simulink model "interp_2D_flat_CLIP_last_index_true"  (R2017b)
settings: Solver=FixedStepAuto  StartTime=0.0  StopTime=10.0  FixedStep=0.1  RelTol=1e-3  EnableMultiTasking=on
settings Model: ExtModeAutoUpdateStatusClock=off  Creator=The MathWorks, Inc.  LastModifiedBy=hbourbou
settings DataIOCC: LimitDataPoints=on  SaveFormat=Array  SignalLoggingName=sigsOut
settings OptimizationCC: BooleanDataType=off  ExpressionDepthLimit=2147483647  InitFltsAndDblsToZero=on  LifeSpan=inf
settings DebuggingCC: SaveWithParameterizedLinksMsg=none  UnderspecifiedInitializationDetection=Classic  MergeDetectMultiDrivingBlocksExec=none  CheckExecutionContextPreStartOutputMsg=on  CheckExecutionContextRuntimeOutputMsg=on  SignalResolutionControl=TryResolveAllWithWarning  MultiTaskDSMMsg=warning  MultiTaskCondExecSysMsg=none  FcnCallInpInsideContextMsg=warning  StateNameClashWarn=warning  SFUnexpectedBacktrackingDiag=warning  SFNoUnconditionalDefaultTransitionDiag=warning  SFExecutionAtInitializationDiag=none
settings HardwareCC: ProdBitPerPointer=32  ProdBitPerSizeT=32  ProdBitPerPtrDiffT=32  ProdLargestAtomicFloat=None  ProdIntDivRoundTo=Undefined  ProdEndianess=Unspecified  ProdWordSize=32  ProdHWDeviceType=32-bit Generic  TargetUnknown=on
settings ModelReferenceCC: PropagateSignalLabelsOutOfModel=off
settings CodeAppCC: StateflowObjectComments=on
settings GRTTargetCC: TargetFcnLib=ansi_tfl_tmw.mat  TargetLangStandard=C89/C90 (ANSI)  GeneratePreprocessorConditionals=Disable all  CombineOutputUpdateFcns=off  GRTInterface=on
settings ConfigComp: CovMetricSettings=dw  CovHtmlReporting=on  CovSaveCumulativeToWorkspaceVar=on  CovSaveSingleToWorkspaceVar=on  CovExternalEMLEnable=off  CovSFcnEnable=off

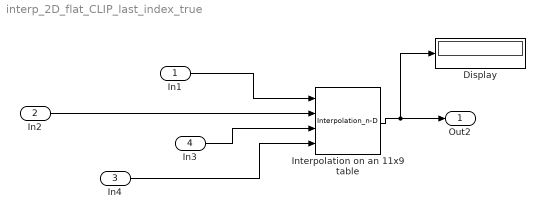
== system interp_2D_flat_CLIP_last_index_true ==
  In1 : Inport  OutMin=0  OutMax=15
  In2 : Inport  Port=2  OutMin=-.5  OutMax=1.7
  In4 : Inport  Port=3  OutMin=-.5  OutMax=1.7
  In3 : Inport  Port=4  OutMin=0  OutMax=15
  Display : Display
  Interpolation on an 11x9 table : Interpolation_n-D  Table=reshape([1:99], [11,9])  InterpMethod=Flat  ExtrapMethod=Clip  ValidIndexMayReachLast=on
  Out2 : Outport
  wires:
  In1/1 -> Interpolation on an 11x9 table/1
  In2/1 -> Interpolation on an 11x9 table/2
  Interpolation on an 11x9 table/1 -> Display/1, Out2/1
  In3/1 -> Interpolation on an 11x9 table/3
  In4/1 -> Interpolation on an 11x9 table/4
